simulink model "trajectoryControllerPlant"  (R2023a)
settings: Solver=VariableStepAuto  StartTime=0.0  StopTime=10.0  RelTol=1e-3
undefined symbols (not defined in the file): data
libraries: sldrtlib x3
settings Model: Creator=fluky  LastModifiedBy=fluky

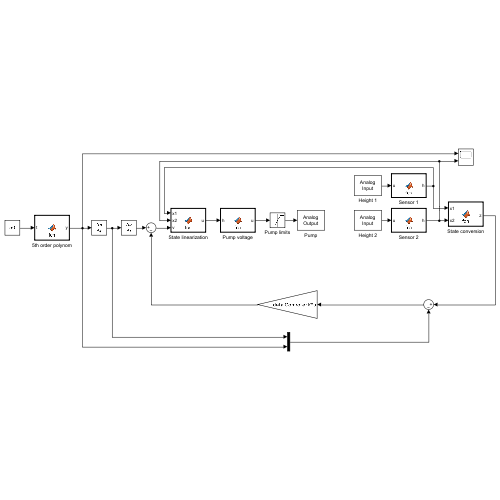
[thumbnail: Simulink's stored preview of the top-level diagram]
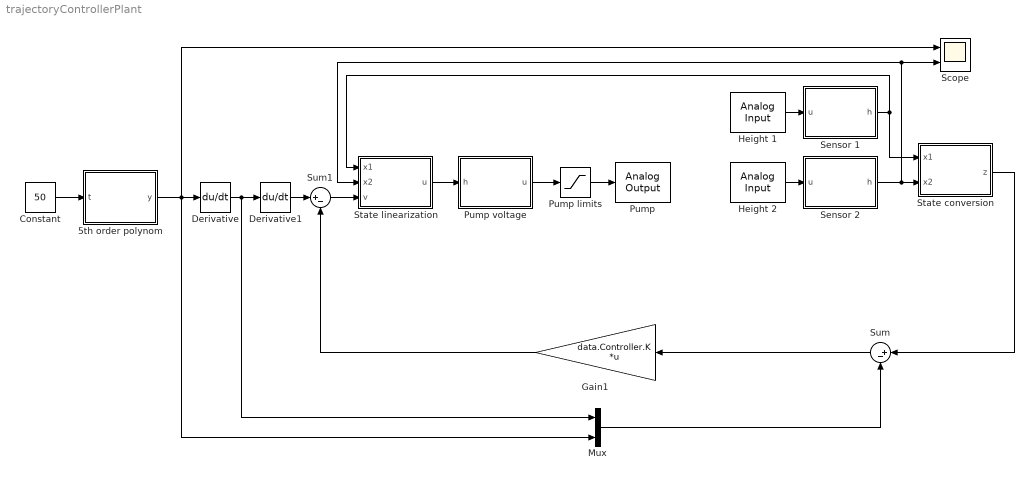
== system trajectoryControllerPlant ==
  5th order polynom : MATLAB Function  TreatAsAtomicUnit=on
  Constant : Constant  Value=50
  Derivative : Derivative
  Derivative1 : Derivative
  Gain1 : Gain  Gain=data.Controller.K  Multiplication=Matrix(K*u)
  Height 1 : sldrtlib/Analog Input  SampleTime=0.1  MaxMissedTicks=10  ShowMissedTicks=off  YieldWhenWaiting=off  DrvAddress=0  DrvOptions=0  Channels=1  RangeMode=1  VoltRange=1  DataType=1
  Height 2 : sldrtlib/Analog Input  SampleTime=0.1  MaxMissedTicks=10  ShowMissedTicks=off  YieldWhenWaiting=off  DrvAddress=0  DrvOptions=0  Channels=1  RangeMode=1  VoltRange=1  DataType=1
  Mux : Mux  Inputs=2
  Pump : sldrtlib/Analog Output  SampleTime=0.1  MaxMissedTicks=10  ShowMissedTicks=off  YieldWhenWaiting=off  DrvAddress=0  DrvOptions=0  Channels=1  RangeMode=1  VoltRange=1  InitialValue=[]  FinalValue=[]
  Pump limits : Saturate  UpperLimit=data.pumpMax  LowerLimit=data.pumpMin
  Pump voltage : MATLAB Function  TreatAsAtomicUnit=on
  Scope : Scope  NumInputPorts=2
  Sensor 1 : MATLAB Function  TreatAsAtomicUnit=on
  Sensor 2 : MATLAB Function  TreatAsAtomicUnit=on
  State conversion : MATLAB Function  TreatAsAtomicUnit=on
  State linearization : MATLAB Function  TreatAsAtomicUnit=on
  Sum : Sum  Inputs=|+-
  Sum1 : Sum  Inputs=|+-
  wires:
  State linearization/1(u) -> Pump voltage/1(h)
  State conversion/1(z) -> Sum/1
  Sum/1 -> Gain1/1
  Sum1/1 -> State linearization/3(v)
  Gain1/1 -> Sum1/2
  Mux/1 -> Sum/2
  Pump limits/1 -> Pump/1
  Pump voltage/1(u) -> Pump limits/1
  Height 1/1 -> Sensor 1/1(u)
  Sensor 2/1(h) -> Scope/2, State linearization/2(x2), State conversion/2(x2)
  Sensor 1/1(h) -> State linearization/1(x1), State conversion/1(x1)
  Height 2/1 -> Sensor 2/1(u)
  Constant/1 -> 5th order polynom/1(t)
  Derivative/1 -> Mux/1, Derivative1/1
  Derivative1/1 -> Sum1/1
  5th order polynom/1(y) -> Mux/2, Scope/1, Derivative/1

== matlab function trajectoryControllerPlant/State conversion ==
  data: x1 input; z output; x2 input; data parameter
function z = fcn(x1, x2, data)

z = [0;0];
z(1) = x2; % is equal to y
z(2) = data.a*sqrt(x1) - data.a*sqrt(x2); % is equal to y_dot

== matlab function trajectoryControllerPlant/State linearization ==
  data: x1 input; u output; x2 input; v input; data parameter
function u = fcn(x1, x2, v, data)

u = data.roh * data.At * sqrt(x1) * (2*v/data.a + data.a * sqrt(x1/x2));

== matlab function trajectoryControllerPlant/5th order polynom ==
  data: t input; y output; data parameter
function y = fcn(t, data)

t = t + 0.0001; % Error otherwise

% Script exp. 5.16
if t <= data.traj.T
    % Trajectory of the system -> smooth at beginning and end
    y = data.traj.y1+(data.traj.y2-data.traj.y1)*(6*(t/data.traj.T)^5-15*(t/data.traj.T)^4+10*(t/data.traj.T)^3);
else
    % End value of the trajectory
    y = data.traj.y2;
end

== matlab function trajectoryControllerPlant/Pump voltage ==
  data: h input; u output; data parameter
function u = fcn(h, data)
% calculation of the pump massflow
u = (h/data.rho + 2125/(210*10^6)) / (3570/(210*10^6));

== matlab function trajectoryControllerPlant/Sensor 1 ==
  data: u input; h output; data parameter
function h = fcn(u, data)
% Height = x1 * voltageSensor + x2 (x1 and x2 from polyfit)
h = data.Sensor.FitPara(1)*u + data.Sensor.FitPara(2)

== matlab function trajectoryControllerPlant/Sensor 2 ==
  data: u input; h output; data parameter
function h = fcn(u, data)
% Height = x1 * voltageSensor + x2 (x1 and x2 from polyfit)
h = data.Sensor.FitPara(1)*u + data.Sensor.FitPara(2)
